simulink model "sim_environment_ltr_gcc"  (Simulink 8.6)
settings: Solver=VariableStepAuto  StartTime=0.0  StopTime=100  RelTol=1e-3
values from neighbouring files (symbols this model uses):
  controller_parameters = struct()    [sim_init.m]
  simulation_parameters = struct()    [sim_init.m]
  vehicle_parameters = struct()    [sim_init.m]
libraries: aerolibactuator x3
settings Model: Creator=cmasserafilho  LastModifiedBy=cmasserafilho
settings DataIOCC: LimitDataPoints=off  SaveFormat=Dataset  SignalLoggingSaveFormat=Dataset  ReturnWorkspaceOutputs=on
settings OptimizationCC: ExpressionDepthLimit=128
settings DebuggingCC: UnderspecifiedInitializationDetection=Simplified  MergeDetectMultiDrivingBlocksExec=error  SolverPrmCheckMsg=none  FcnCallInpInsideContextMsg=EnableAllAsError  StateNameClashWarn=none
settings HardwareCC: ProdBitPerPointer=64  ProdLargestAtomicFloat=Float  ProdIntDivRoundTo=Zero  ProdEndianess=LittleEndian  ProdWordSize=64  ProdHWDeviceType=Intel->x86-64 (Windows64)
settings GRTTargetCC: GeneratePreprocessorConditionals=Use local settings  CombineOutputUpdateFcns=on  GRTInterface=off
settings ConfigComp: CovModelRefEnable=off

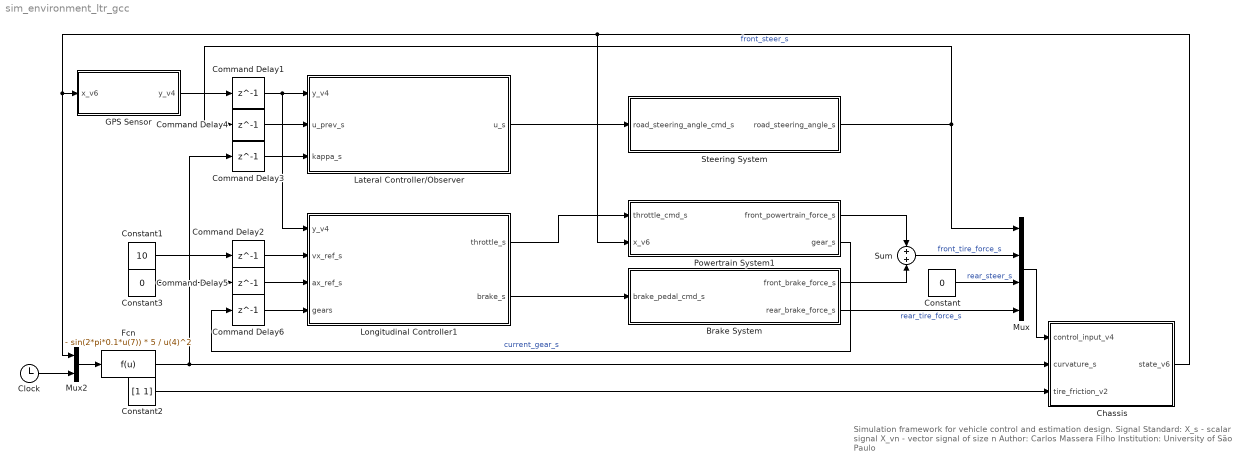
== system sim_environment_ltr_gcc ==
  note: Simulation framework for vehicle control and estimation design.
      |
      | Signal Standard:
      | X_s - scalar signal
      | X_vn - vector signal of size n
      |
      | Author: Carlos Massera Filho
      | Institution: University of São Paulo
  Brake System : Subsystem
  Chassis : Subsystem
  Clock : Clock
  Command Delay{1..6} (6 alike) : Delay  DelayLength=1  InitialCondition=0  SampleTime=controller_parameters.Ts
  Constant : Constant  Value=0
  Constant1 : Constant  Value=10
  Constant2 : Constant  Value=[1 1]
  Constant3 : Constant  Value=0
  Fcn : Fcn  Expr=- sin(2*pi*0.1*u(7)) * 5 / u(4)^2
  GPS Sensor : MATLAB Function  TreatAsAtomicUnit=on
  Lateral Controller/Observer : Subsystem
  Longitudinal Controller1 : Subsystem
  Mux : Mux
  Mux2 : Mux  Inputs=2
  Powertrain System1 : Subsystem
  Steering System : Subsystem
  Sum : Sum  Inputs=+|+
  wires:
  Chassis/1(state_v6) -> Powertrain System1/2(x_v6), Mux2/1, GPS Sensor/1(x_v6)
  Mux/1 -> Chassis/1(control_input_v4)
  Constant/1 -> Mux/3  "rear_steer_s"
  Sum/1 -> Mux/2  "front_tire_force_s"
  Brake System/2(rear_brake_force_s) -> Mux/4  "rear_tire_force_s"
  Brake System/1(front_brake_force_s) -> Sum/2
  Powertrain System1/1(front_powertrain_force_s) -> Sum/1
  Steering System/1("road_steering_angle_s ") -> Mux/1, Command Delay4/1  "front_steer_s"
  Constant2/1 -> Chassis/3(tire_friction_v2)
  Fcn/1 -> Chassis/2(curvature_s), Command Delay3/1
  Mux2/1 -> Fcn/1
  Clock/1 -> Mux2/2
  Command Delay4/1 -> Lateral Controller/Observer/2(u_prev_s)
  Command Delay3/1 -> Lateral Controller/Observer/3(kappa_s)
  Lateral Controller/Observer/1(u_s) -> Steering System/1(road_steering_angle_cmd_s)
  Command Delay1/1 -> Longitudinal Controller1/1(y_v4), Lateral Controller/Observer/1(y_v4)
  GPS Sensor/1(y_v4) -> Command Delay1/1
  Longitudinal Controller1/2(brake_s) -> Brake System/1(brake_pedal_cmd_s)
  Longitudinal Controller1/1(throttle_s) -> Powertrain System1/1(throttle_cmd_s)
  Command Delay2/1 -> Longitudinal Controller1/2(vx_ref_s)
  Command Delay5/1 -> Longitudinal Controller1/3(ax_ref_s)
  Constant1/1 -> Command Delay2/1
  Constant3/1 -> Command Delay5/1
  Powertrain System1/2(gear_s) -> Command Delay6/1  "current_gear_s"
  Command Delay6/1 -> Longitudinal Controller1/4(gears)

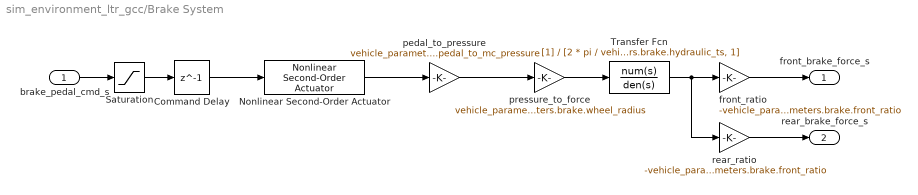
== system sim_environment_ltr_gcc/Brake System ==
  brake_pedal_cmd_s : Inport
  Command Delay : Delay  DelayLength=1  InitialCondition=0  SampleTime=vehicle_parameters.brake.delay
  Nonlinear Second-Order Actuator : aerolibactuator/Nonlinear Second-Order Actuator  wn_fin=2 * pi / vehicle_parameters.brake.actuator_tc  z_fin=1  fin_max=1  fin_min=0  fin_maxrate=vehicle_parameters.brake.rate_limit  fin_act_0=0  fin_act_vel=0
  Saturation : Saturate  UpperLimit=1  LowerLimit=0
  Transfer Fcn : TransferFcn  Denominator=[2 * pi / vehicle_parameters.brake.hydraulic_ts, 1]
  front_ratio : Gain  Gain=-vehicle_parameters.brake.front_ratio
  pedal_to_pressure : Gain  Gain=vehicle_parameters.brake.pedal_to_mc_pressure
  pressure_to_force : Gain  Gain=vehicle_parameters.brake.mc_pressure_to_torque / vehicle_parameters.brake.wheel_radius
  rear_ratio : Gain  Gain=-vehicle_parameters.brake.front_ratio
  front_brake_force_s : Outport
  rear_brake_force_s : Outport  Port=2
  wires:
  brake_pedal_cmd_s/1 -> Saturation/1
  front_ratio/1 -> front_brake_force_s/1
  rear_ratio/1 -> rear_brake_force_s/1
  Saturation/1 -> Command Delay/1
  Nonlinear Second-Order Actuator/1 -> pedal_to_pressure/1
  Command Delay/1 -> Nonlinear Second-Order Actuator/1
  pressure_to_force/1 -> Transfer Fcn/1
  Transfer Fcn/1 -> rear_ratio/1, front_ratio/1
  pedal_to_pressure/1 -> pressure_to_force/1

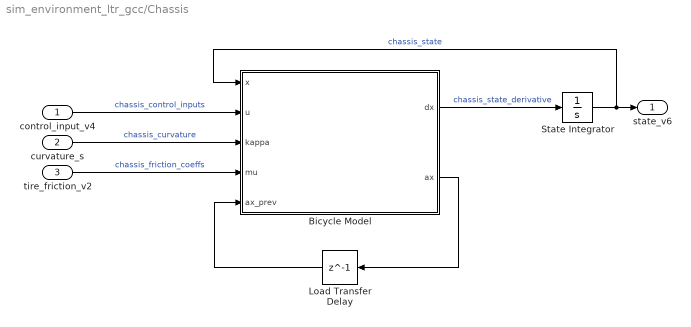
== system sim_environment_ltr_gcc/Chassis ==
  control_input_v4 : Inport
  curvature_s : Inport  Port=2
  tire_friction_v2 : Inport  Port=3
  Bicycle Model : MATLAB Function  TreatAsAtomicUnit=on
  Load Transfer Delay : Delay  DelayLength=1  InitialCondition=0  SampleTime=vehicle_parameters.uncertainty.load_transfer_Ts
  State Integrator : Integrator  InitialCondition=simulation_parameters.x0
  state_v6 : Outport
  wires:
  control_input_v4/1 -> Bicycle Model/2(u)  "chassis_control_inputs"
  State Integrator/1 -> state_v6/1, Bicycle Model/1(x)  "chassis_state"
  Load Transfer Delay/1 -> Bicycle Model/5(ax_prev)
  curvature_s/1 -> Bicycle Model/3(kappa)  "chassis_curvature"
  Bicycle Model/2(ax) -> Load Transfer Delay/1
  Bicycle Model/1(dx) -> State Integrator/1  "chassis_state_derivative"
  tire_friction_v2/1 -> Bicycle Model/4(mu)  "chassis_friction_coeffs"

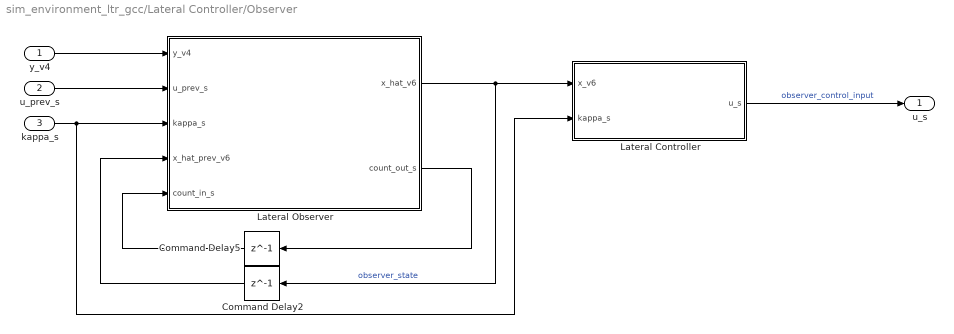
== system sim_environment_ltr_gcc/Lateral Controller/Observer ==
  y_v4 : Inport
  u_prev_s : Inport  Port=2
  kappa_s : Inport  Port=3
  Command Delay2 : Delay  DelayLength=1  InitialCondition=0  SampleTime=controller_parameters.Ts
  Command Delay5 : Delay  DelayLength=1  InitialCondition=0  SampleTime=controller_parameters.Ts
  Lateral Controller : MATLAB Function  TreatAsAtomicUnit=on
  Lateral Observer : MATLAB Function  TreatAsAtomicUnit=on
  u_s : Outport
  wires:
  Lateral Controller/1(u_s) -> u_s/1  "observer_control_input"
  Command Delay2/1 -> Lateral Observer/4(x_hat_prev_v6)
  Lateral Observer/1(x_hat_v6) -> Command Delay2/1, Lateral Controller/1(x_v6)  "observer_state"
  kappa_s/1 -> Lateral Observer/3(kappa_s), Lateral Controller/2(kappa_s)
  y_v4/1 -> Lateral Observer/1(y_v4)
  u_prev_s/1 -> Lateral Observer/2(u_prev_s)
  Lateral Observer/2(count_out_s) -> Command Delay5/1
  Command Delay5/1 -> Lateral Observer/5(count_in_s)

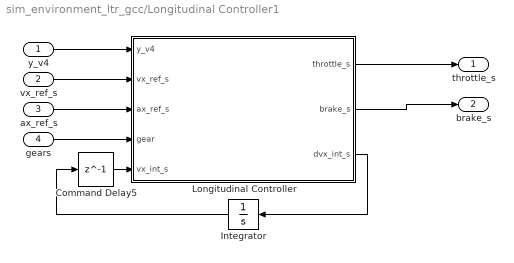
== system sim_environment_ltr_gcc/Longitudinal Controller1 ==
  y_v4 : Inport
  vx_ref_s : Inport  Port=2
  ax_ref_s : Inport  Port=3
  gears : Inport  Port=4
  Command Delay5 : Delay  DelayLength=1  InitialCondition=0  SampleTime=controller_parameters.Ts
  Integrator : Integrator
  Longitudinal Controller : MATLAB Function  TreatAsAtomicUnit=on
  throttle_s : Outport
  brake_s : Outport  Port=2
  wires:
  y_v4/1 -> Longitudinal Controller/1(y_v4)
  Integrator/1 -> Command Delay5/1
  Longitudinal Controller/3(dvx_int_s) -> Integrator/1
  vx_ref_s/1 -> Longitudinal Controller/2(vx_ref_s)
  ax_ref_s/1 -> Longitudinal Controller/3(ax_ref_s)
  Longitudinal Controller/2(brake_s) -> brake_s/1
  Longitudinal Controller/1(throttle_s) -> throttle_s/1
  Command Delay5/1 -> Longitudinal Controller/5(vx_int_s)
  gears/1 -> Longitudinal Controller/4(gear)

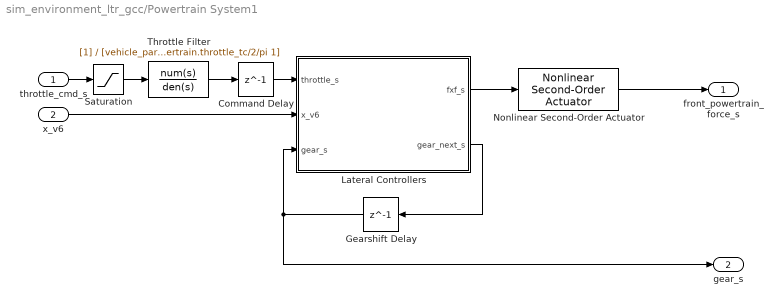
== system sim_environment_ltr_gcc/Powertrain System1 ==
  throttle_cmd_s : Inport
  x_v6 : Inport  Port=2
  Command Delay : Delay  DelayLength=1  InitialCondition=0  SampleTime=vehicle_parameters.powertrain.delay
  Gearshift Delay : Delay  DelayLength=1  InitialCondition=0  SampleTime=vehicle_parameters.powertrain.gear_shift_delay
  Lateral Controllers : MATLAB Function  TreatAsAtomicUnit=on
  Nonlinear Second-Order Actuator : aerolibactuator/Nonlinear Second-Order Actuator  wn_fin=2 * pi / vehicle_parameters.powertrain.engine_tc  z_fin=1  fin_max=Inf  fin_min=-Inf  fin_maxrate=Inf  fin_act_0=0  fin_act_vel=0
  Saturation : Saturate  UpperLimit=1  LowerLimit=0
  Throttle Filter : TransferFcn  Denominator=[vehicle_parameters.powertrain.throttle_tc/2/pi 1]
  front_powertrain_force_s : Outport
  gear_s : Outport  Port=2
  wires:
  Lateral Controllers/1(fxf_s) -> Nonlinear Second-Order Actuator/1
  throttle_cmd_s/1 -> Saturation/1
  Throttle Filter/1 -> Command Delay/1
  Lateral Controllers/2(gear_next_s) -> Gearshift Delay/1
  Gearshift Delay/1 -> Lateral Controllers/3(gear_s), gear_s/1
  Nonlinear Second-Order Actuator/1 -> front_powertrain_force_s/1
  x_v6/1 -> Lateral Controllers/2(x_v6)
  Command Delay/1 -> Lateral Controllers/1(throttle_s)
  Saturation/1 -> Throttle Filter/1

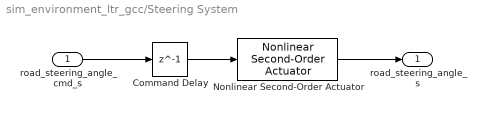
== system sim_environment_ltr_gcc/Steering System ==
  road_steering_angle_cmd_s : Inport
  Command Delay : Delay  DelayLength=1  InitialCondition=0  SampleTime=vehicle_parameters.steering.delay
  Nonlinear Second-Order Actuator : aerolibactuator/Nonlinear Second-Order Actuator  wn_fin=2 * pi / vehicle_parameters.steering.tc  z_fin=1  fin_max=vehicle_parameters.steering.angle_limit  fin_min=-vehicle_parameters.steering.angle_limit  fin_maxrate=vehicle_parameters.steering.rate_limit  fin_act_0=0  fin_act_vel=0
  "road_steering_angle_s " : Outport
  wires:
  road_steering_angle_cmd_s/1 -> Command Delay/1
  Command Delay/1 -> Nonlinear Second-Order Actuator/1
  Nonlinear Second-Order Actuator/1 -> "road_steering_angle_s "/1

== matlab function Lateral Controller//Observer/Lateral Controller ==
  data: x_v6 input double; u_s output double; kappa_s input double; controller parameter double
function u_s = lateral_control_wrapper(x_v6, kappa_s, controller)

    u_s = lateral_control(x_v6, kappa_s, controller.lateral);
    
end

== matlab function Chassis/Bicycle Model ==
  data: x input double; u input double size=4; dx output double; kappa input double; mu input double; ax_prev input double; vehicle_parameters parameter double; ax output double
function [dx, ax] = bicycle_model_wrapper(x, u, kappa, mu, ax_prev, vehicle_parameters)

    [dx, ax] = nonliear_bicycle_model(x, u, kappa, mu, ax_prev, vehicle_parameters);
    
end

== matlab function Lateral Controller//Observer/Lateral Observer ==
  data: y_v4 input double; u_prev_s input double; kappa_s input double; observer parameter double; x_hat_prev_v6 input double; x_hat_v6 output double; count_in_s input double; count_out_s output double
function [x_hat_v6, count_out_s] = lateral_observer_wrapper(y_v4, u_prev_s, kappa_s, observer, x_hat_prev_v6, count_in_s)

    x_hat_v6 = zeros(6,1);
    count_out_s = 0;
    
    x_hat_v6 = lateral_observer(y_v4, x_hat_prev_v6, u_prev_s, kappa_s, observer, count_in_s == 0);
    
    count_out_s = mod(count_in_s + 1, observer.subsampling);
end

== matlab function GPS Sensor ==
  data: x_v6 input double; y_v4 output double; simulation_parameters parameter double
function y_v4 = gps_sensor_wrapper(x_v6, simulation_parameters)

    y_v4 = zeros(size(simulation_parameters.gps.C, 1),1);
    y_v4 = gps_sensor(x_v6, simulation_parameters);
    
end

== matlab function Longitudinal Controller1/Longitudinal Controller ==
  data: y_v4 input double; throttle_s output double; vx_ref_s input double; ax_ref_s input double; gear input double; vx_int_s input double; controller parameter double; brake_s output double; dvx_int_s output double
function [throttle_s, brake_s, dvx_int_s] = longitudinal_control_wrapper(y_v4, vx_ref_s, ...
                                                                         ax_ref_s, gear, ...
                                                                         vx_int_s, controller)

    [throttle_s, brake_s, dvx_int_s] = longitudinal_control(y_v4(3), vx_ref_s, ax_ref_s, ...
                                                            vx_int_s, gear, ...
                                                            controller.longitudinal);
    
end

== matlab function Powertrain System1/Lateral Controllers ==
  data: throttle_s input double; x_v6 input double; gear_s input double; fxf_s output double; vehicle_parameters parameter double; gear_next_s output double
function [fxf_s, gear_next_s] = powertrain_model_wrapper(throttle_s, x_v6, gear_s, vehicle_parameters)

    [fxf_s, gear_next_s] = powertrain_model(throttle_s, x_v6, gear_s, vehicle_parameters.powertrain);
    
end
